simulink model "Motion_planner_Street_Drone"  (R2019b)
settings: Solver=FixedStepAuto  StartTime=0.0  StopTime=25  FixedStep=0.0075  MaxStep=1e-1  MinStep=1e-3  RelTol=1e-3  AbsTol=1e-4
InitFcn:
  | SD_init1
values from neighbouring files (symbols this model uses):
  cost = [2.71432892747 3.32441927977 3.79268757264 4.85642115368 6.12135035287 7.09825974303 9.57278659789 1.55754789407 1.51399555616 2.57723707661 3.8468529147 4.8336387623 ... (2430 elements, 1x2430)]    [matlab.mat]
  Front_brake = [0 2.2085352751 4.15209150797 6.12733711785 8.16604105928 9.79119154879 12.1808659635 14.1242630413 16.1155522836 18.1386900579 20.0839213981 22.1313006548 ... (68 elements, 34x2)]    [Front_brake.mat]
  N = size(X,1)    [curvature.m]
  obsx = [dx1 dx2 dx3 dx4]'    [dynamic_collison.m]    (also in dynamic_detection1.m = [x1 x2 x3 x4]')
  obsy = [dy1 dy2 dy3 dy4]'    [dynamic_collison.m]    (also in dynamic_detection1.m = [y1 y2 y3 y4]')
  x = obs_path(i,1)    [dynamic_collison.m]    (also in dynamic_detection1.m)
  X = [X]    [curvature.m]
  y = obs_path(i,2)    [dynamic_collison.m]    (also in dynamic_detection1.m)
undefined symbols (not defined in the file or in its folder): d, dfin, dini, Ki, Kp, L_0f, lookahead_time, lookahead_time_rev, Rear_brake, sigbuilder_block, steer_ratio, steer_sens, tfin, tini, TPS_0, xfin, Y, yfin, Z
libraries: sm_lib x290, nesl_utility x136, simulink x6, vrlib x2, powerlib_meascontrol x2
(part 14 of 14)

== matlab function Motion_planner_Street_Drone/Descision_layer/Subsystem/MATLAB Function2 ==
  data: xa input; mode1 output; ya input; ta input; park_goal input; Vin input; mode input; new output; path input; x_i output; y_i output; t_i output; obsc output; vel_in output; v2 output; switch1 output; AEB output
function [mode1,new,x_i,y_i,t_i,obsc,vel_in,v2,switch1,AEB]= fcn(xa,ya,ta,park_goal,Vin, mode, path)
coder.extrinsic('InPolygon')
%this function is to check the static obstacle, replanning, parking spot detection,
%emergency braking

switch1=1;
v2=1;
mode1=mode;
new=0;
cur =   struct('xa',0,'ya',0);
x_i=xa;
y_i=ya;
t_i=ta;
AEB=1;
obsc=2;
vel_in=Vin;
 select = ~isnan(path(:,1));
path1=path(select,(1:4));
path_inputx=path1(:,1);
path_inputy=path1(:,2);
path_inputtf=path1(:,3);
obst_check=1;
% Please put the obstacle in the path with most number of vertices as the first obstacle.
%(same as mention in SD_init1.m
obsx= [85,88,88,85];
obsy = [-1.2,-1.2,1.2,1.2];

  cur.xa=xa;
   cur.ya=ya;
   cur.t=ta;
%% Emergency Braking
 Emergency_brake = Emergency_braking(cur,obsx,obsy,1);
 if Emergency_brake==true
          AEB=-1;
  else
         AEB=1;
 end
  % Static obstacle Detection
    obs_inside_window = check_for_obs(cur,obsx,obsy,1);
    
if obs_inside_window==true
        %disp('obstacle')
        
       xp=path_inputx;
       yp=path_inputy;
       thetap=path_inputtf;
       cur.xa=0;
       cur.ya=0;
obsx= [85,87,87,85];
obsy = [-1.2,-1.2,1.2,1.2];
      obst_check = obs_check(cur,xp,yp,thetap,0,1,1,obsx,obsy);
        
       if obst_check==0
           obsc=3;
           new=1 ;
%            x_i=xa;
%            y_i=ya;
%            t_i=0;
        
         
         vel_in=Vin;
        
          return
       end

   return
end    
 
%% Parking spot detection
%  if 80<xa && xa<100 && mode==2
% % % Angle of the vectors
%  oh_f = 2.1;  % Longitudinal distance from the rear axle to the front of the vehicle [m]
%  w_1   = 18;     % Width of vehicle [m]
%  lv34_1 = hypot((w_1/2),oh_f); % Length of Vector 3 and 4
% vmax=2.78;
% 
%  switch1=-1;
% % % 
% % % 
%   %v2=sqrt(complex((2*(-1)*((xa-80)))+(vmax)^2));
%   %v2=max(real(v2),0.5);
%  av3 = (180/pi*ta)-atand((w_1/2)/oh_f); % Angle of Vector 3
%  av4 = (180/pi*ta)+atand((w_1/2)/oh_f); % Angle of Vector 4
% % 
% % % Finding the actual points
%  xv1_1 = xa;
%  yv1_1 = ya;
%  xv3_1 = lv34_1*cosd(av3)+xa;
%  yv3_1 = lv34_1*sind(av3)+ya;
%  xv4_1 = lv34_1*cosd(av4)+xa;
%  yv4_1 = lv34_1*sind(av4)+ya;
% % 
% % 
%  xc=[xv1_1;xv3_1;xv4_1];
%  yc=[yv1_1;yv3_1;yv4_1];
% % i=1
% %        streetdrone= polyshape([xc(i,1);xc(i,2);xc(i,3)],[yc(i,1);yc(i,2);yc(i,3)]);
% % %           
% %       axis equal;
% %             plot(streetdrone);
%      %%
%          in12=zeros(1, 'logical');
%         in12 = inpolygon(park_goal(1),park_goal(2),xc,yc); % check whether cur is hitting obs
%         in12 = any(in12);
%          if in12 == 1 && mode==2
%          mode1=3;
%          v2=0;
%          vel_in=0;
%          new=1;
%          end
  end

== matlab function Motion_planner_Street_Drone/Trajectory Tracker/Longitudinal Controller/MATLAB Function ==
  data: ux input; y output; uy input; t input
function y = fcn(ux,uy,t)

y = ux*cos(t)-uy*sin(t);

== matlab function Motion_planner_Street_Drone/Dynamic_Obstacle_avoidance/Subsystem2/HOLD ==
  settings: updateMethod=DISCRETE
  data: u input; y output

function y = fcn(u)
  persistent flag
  if isempty(flag)
     flag = true;
  end
  if flag
     y = u;
     if u==-1
        flag = false;
     end
  else
     y = -1;
  end
end

== matlab function Motion_planner_Street_Drone/Dynamic_Obstacle_avoidance/Subsystem2/Stop & GO ==
  data: stopx input; stopy input; stop output; x input; y input
function stop  = fcn(stopx,stopy, x,y)
%to stop the vehicle to pass the dynamic obstacle
if abs(stopx(1,1)-x)<0.1 && abs(stopy-y)<0.01
   stop=1;
else
   stop=0;
end

== stateflow chart Motion_planner_Street_Drone/Dynamic_Obstacle_avoidance/Subsystem2/Chart1 ==
  state Forward
    y=0;
  state Neutral
    y=-1;
  (default) -> Forward
  Forward -> Neutral : [stop==1]
  Neutral -> Forward : after (6,sec)
  data: y output; stop input

== stateflow chart Motion_planner_Street_Drone/Goal_check/Chart1 ==
  state Forward
    y=1;
    y1=0;
    mode=1;
  state Neutral
    y=0;
    y1=1;
    mode=1;
  state Neutral1
    stop=0;
  (default) -> Forward
  Forward -> Neutral : [goal==1]
  Neutral -> Neutral1 : [goal==1]
  data: y output; goal input; y1 output; mode output; stop output
